simulink model "model1_analysis_trial_descf"  (R2022a)
settings: Solver=VariableStepAuto  StartTime=0.0  StopTime=50  RelTol=1e-3
undefined symbols (not defined in the file): Kc, Kd, Ki, Kp
settings Model: Creator=srika  LastModifiedBy=srika

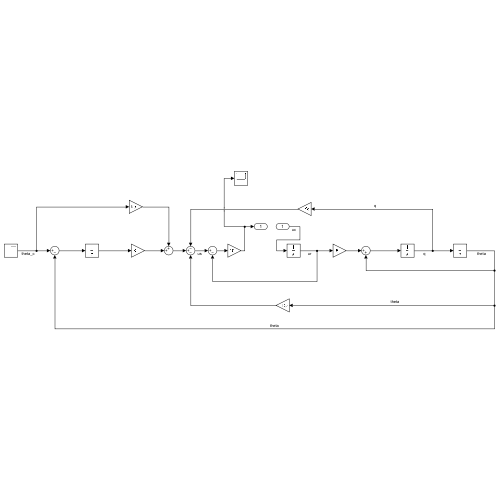
[thumbnail: Simulink's stored preview of the top-level diagram]
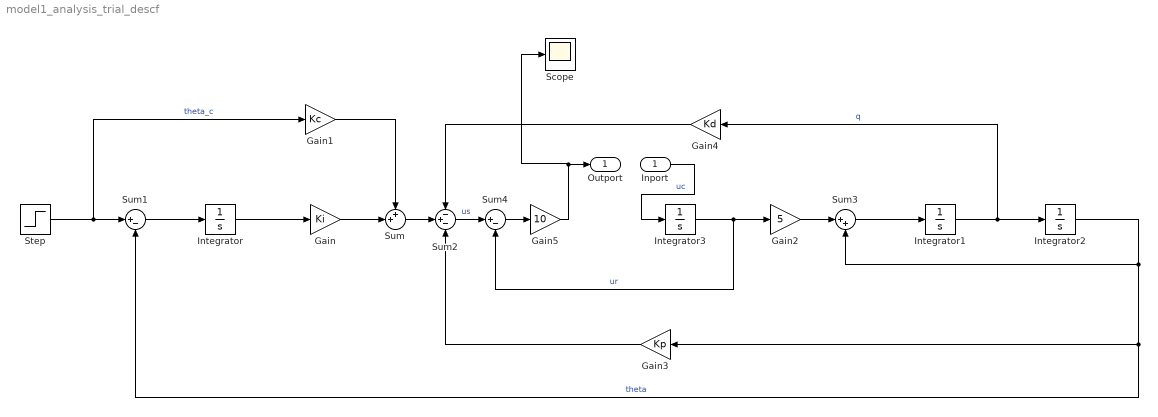
== system model1_analysis_trial_descf ==
  Inport : Inport
  Gain : Gain  Gain=Ki
  Gain1 : Gain  Gain=Kc
  Gain2 : Gain  Gain=5
  Gain3 : Gain  Gain=Kp
  Gain4 : Gain  Gain=Kd
  Gain5 : Gain  Gain=10
  Integrator{,1..3} (4 alike) : Integrator
  Scope : Scope
  Step : Step  Time=0  After=0.3879  SampleTime=0
  Sum : Sum  Inputs=++|
  Sum1 : Sum  Inputs=|+-
  Sum2 : Sum  Inputs=-+-
  Sum3 : Sum  Inputs=|++
  Sum4 : Sum  Inputs=|+-
  Outport : Outport
  wires:
  Step/1 -> Gain1/1, Sum1/1  "theta_c"
  Sum1/1 -> Integrator/1
  Integrator/1 -> Gain/1
  Gain/1 -> Sum/2
  Gain1/1 -> Sum/1
  Sum/1 -> Sum2/2
  Integrator3/1 -> Gain2/1, Sum4/2  "ur"
  Gain2/1 -> Sum3/1
  Sum3/1 -> Integrator1/1
  Integrator1/1 -> Gain4/1, Integrator2/1  "q"
  Integrator2/1 -> Sum1/2, Gain3/1, Sum3/2  "theta"
  Gain3/1 -> Sum2/3
  Gain4/1 -> Sum2/1
  Inport/1 -> Integrator3/1  "uc"
  Sum2/1 -> Sum4/1  "us"
  Sum4/1 -> Gain5/1
  Gain5/1 -> Outport/1, Scope/1
